simulink model "Hp"  (R2017a)
settings: Solver=VariableStepAuto  StartTime=0.0  StopTime=10.0  RelTol=1e-3
libraries: simulink x1
settings Model: Creator=zolubas  LastModifiedBy=zolubas

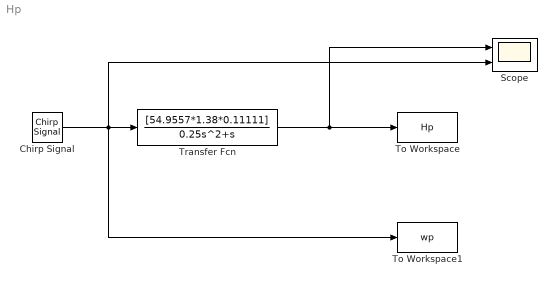
== system Hp ==
  Chirp Signal : simulink/Sources/Chirp Signal  f1=0  T=10  f2=100
  Scope : Scope  NumInputPorts=2
  To Workspace : ToWorkspace  VariableName=Hp  SampleTime=-1
  To Workspace1 : ToWorkspace  VariableName=wp  SampleTime=-1
  Transfer Fcn : TransferFcn  Numerator=[54.9557*1.38*0.11111]  Denominator=[0.25 1 0]
  wires:
  Chirp Signal/1 -> Scope/2, To Workspace1/1, Transfer Fcn/1
  Transfer Fcn/1 -> Scope/1, To Workspace/1
